simulink model "DigitalControlProblem"  (R2013b)
settings: Solver=ode45  StartTime=0.0  StopTime=10.0  RelTol=1e-3
libraries: simulink x1
settings Model: Creator=gyurse  LastModifiedBy=gyurse

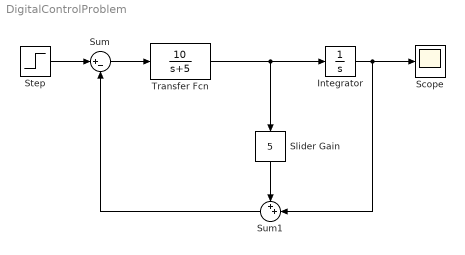
== system DigitalControlProblem ==
  Integrator : Integrator
  Scope : Scope
  Slider Gain : simulink/Math Operations/Slider Gain  low=0  gain=5  high=5
  Step : Step  SampleTime=0
  Sum : Sum  Inputs=|+-
  Sum1 : Sum  Inputs=++|
  Transfer Fcn : TransferFcn  Numerator=[10]  Denominator=[1 5]
  wires:
  Step/1 -> Sum/1
  Transfer Fcn/1 -> Integrator/1, Slider Gain/1
  Sum/1 -> Transfer Fcn/1
  Slider Gain/1 -> Sum1/1
  Integrator/1 -> Scope/1, Sum1/2
  Sum1/1 -> Sum/2
